simulink model "W3_Problem_1"  (R2020a)
settings: Solver=VariableStepAuto  StartTime=0.0  StopTime=10.0  RelTol=1e-3
settings Model: Creator=user  LastModifiedBy=user

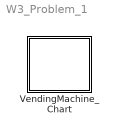
== system W3_Problem_1 ==
  VendingMachine_Chart : Stateflow chart  TreatAsAtomicUnit=on

== stateflow chart W3_Problem_1/VendingMachine_Chart ==
  settings: stateMachineType=MEALY_MACHINE
